simulink model "msim"  (R2024b)
settings: Solver=VariableStepAuto  StartTime=0.0  StopTime=20  RelTol=1e-3
values from neighbouring files (symbols this model uses):
  dirsorder = [11 12]    [main.m]
  MomReg = MomPI(tflin)    [main.m]
  NaslinReg = NaslinPI(tflin, alpha)    [main.m]
  tflin = tf(num, den)    [disc.m]    (also in main.m)
  z = -0.1    [main.m]
settings Model: Creator=markminerov  LastModifiedBy=markminerov

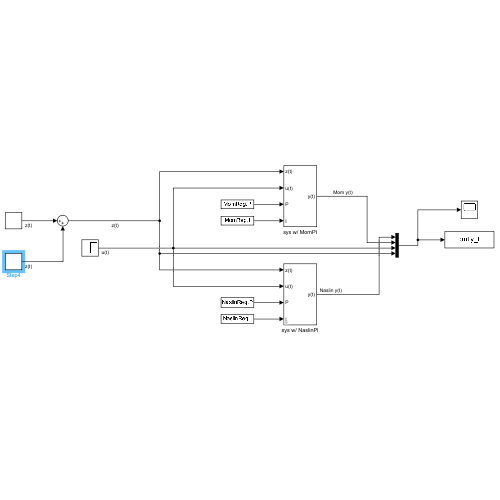
[thumbnail: Simulink's stored preview of the top-level diagram]
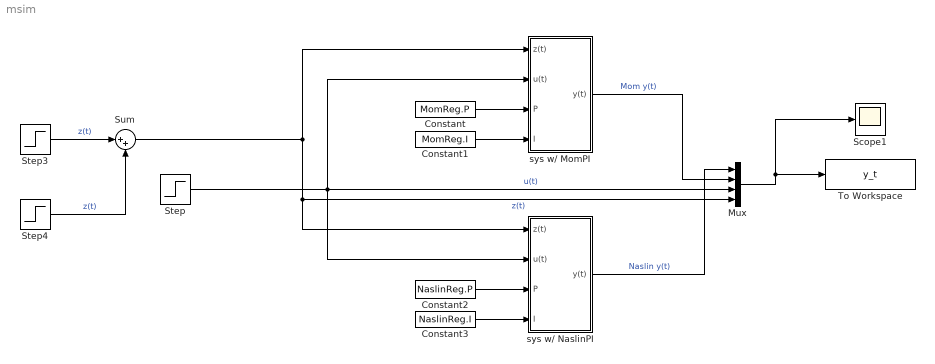
== system msim ==
  Constant : Constant  Value=MomReg.P
  Constant1 : Constant  Value=MomReg.I
  Constant2 : Constant  Value=NaslinReg.P
  Constant3 : Constant  Value=NaslinReg.I
  Mux : Mux
  Scope1 : Scope
  Step : Step  After=u  SampleTime=0
  Step3 : Step  Time=dirsorder(1)  After=z  SampleTime=0
  Step4 : Step  Time=dirsorder(2)  After=-z  SampleTime=0
  Sum : Sum  Inputs=|++
  To Workspace : ToWorkspace  VariableName=y_t  SaveFormat=Timeseries  SampleTime=-1
  sys w/ MomPI : Subsystem
  sys w/ NaslinPI : Subsystem
  wires:
  sys w/ MomPI/1(y(t)) -> Mux/2  "Mom y(t)"
  Constant/1 -> sys w/ MomPI/3(P)
  Constant1/1 -> sys w/ MomPI/4(I)
  Constant3/1 -> sys w/ NaslinPI/4(I)
  Constant2/1 -> sys w/ NaslinPI/3(P)
  Sum/1 -> sys w/ MomPI/1(z(t)), sys w/ NaslinPI/1(z(t)), Mux/4  "z(t)"
  Step/1 -> sys w/ MomPI/2(u(t)), Mux/3, sys w/ NaslinPI/2(u(t))  "u(t)"
  Mux/1 -> Scope1/1, To Workspace/1
  sys w/ NaslinPI/1(y(t)) -> Mux/1  "Naslin y(t)"
  Step3/1 -> Sum/1  "z(t)"
  Step4/1 -> Sum/2  "z(t)"

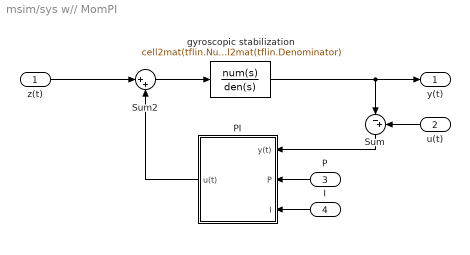
== system msim/sys w// MomPI ==
  z(t) : Inport
  u(t) : Inport  Port=2
  P : Inport  Port=3
  I : Inport  Port=4
  PI : Subsystem
  Sum : Sum  Inputs=|-+
  Sum2 : Sum  Inputs=|++
  gyroscopic stabilization : TransferFcn  Numerator=cell2mat(tflin.Numerator)  Denominator=cell2mat(tflin.Denominator)
      mask Display: image('img.jpg');
  y(t) : Outport
  wires:
  gyroscopic stabilization/1 -> y(t)/1, Sum/1
  Sum2/1 -> gyroscopic stabilization/1
  u(t)/1 -> Sum/2
  Sum/1 -> PI/1(y(t))
  PI/1(u(t)) -> Sum2/2
  z(t)/1 -> Sum2/1
  P/1 -> PI/2(P)
  I/1 -> PI/3(I)

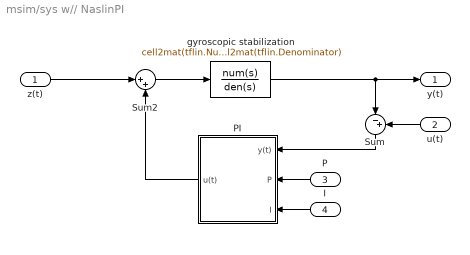
== system msim/sys w// NaslinPI ==
  z(t) : Inport
  u(t) : Inport  Port=2
  P : Inport  Port=3
  I : Inport  Port=4
  PI : Subsystem
  Sum : Sum  Inputs=|-+
  Sum2 : Sum  Inputs=|++
  gyroscopic stabilization : TransferFcn  Numerator=cell2mat(tflin.Numerator)  Denominator=cell2mat(tflin.Denominator)
      mask Display: image('img.jpg');
  y(t) : Outport
  wires:
  gyroscopic stabilization/1 -> y(t)/1, Sum/1
  Sum2/1 -> gyroscopic stabilization/1
  u(t)/1 -> Sum/2
  Sum/1 -> PI/1(y(t))
  PI/1(u(t)) -> Sum2/2
  z(t)/1 -> Sum2/1
  P/1 -> PI/2(P)
  I/1 -> PI/3(I)

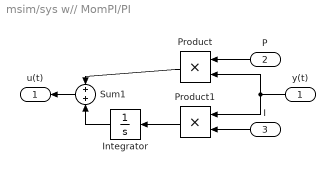
== system msim/sys w// MomPI/PI ==
  y(t) : Inport
  P : Inport  Port=2
  I : Inport  Port=3
  Integrator : Integrator
  Product : Product
  Product1 : Product
  Sum1 : Sum  Inputs=+|+
  u(t) : Outport
  wires:
  y(t)/1 -> Product1/1, Product/2
  Sum1/1 -> u(t)/1
  Product/1 -> Sum1/1
  P/1 -> Product/1
  I/1 -> Product1/2
  Product1/1 -> Integrator/1
  Integrator/1 -> Sum1/2

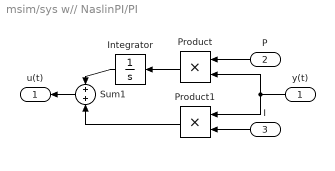
== system msim/sys w// NaslinPI/PI ==
  y(t) : Inport
  P : Inport  Port=2
  I : Inport  Port=3
  Integrator : Integrator
  Product : Product
  Product1 : Product
  Sum1 : Sum  Inputs=+|+
  u(t) : Outport
  wires:
  y(t)/1 -> Product1/1, Product/2
  Sum1/1 -> u(t)/1
  Integrator/1 -> Sum1/1
  Product1/1 -> Sum1/2
  Product/1 -> Integrator/1
  P/1 -> Product/1
  I/1 -> Product1/2
